simulink model "c_ff_pvcm_2dof_ax1_2"  (R2024b)
settings: Solver=VariableStepAuto  StartTime=0.0  StopTime=10.0  RelTol=1e-3
values from neighbouring files (symbols this model uses):
  Ct = 2.0e8    (= 200000000)    [check_2dof_model.m]    (also in ex9.m = 210000000; load_ex9_model.m)
  Dr = 0    [check_2dof_model.m]    (also in ex8_4.m; ex9.m; load_ex9_model.m)
  FBtype = 1    [check_2dof_model.m]    (also in ex8_4.m; ex9.m = -1; load_ex9_model.m)
  Jr = 3.0e-2    (= 0.03)    [check_2dof_model.m]    (also in ex9.m; load_ex9_model.m; load_params.m = 0.00222)
  Kpp = 40    [check_2dof_model.m]    (also in ex8_4.m = 4; ex9.m; load_ex9_model.m)
  KT = 1    [check_2dof_model.m]    (also in ex8_4.m; ex9.m; load_ex9_model.m)
  Kt = 1.0e8    (= 100000000)    [check_2dof_model.m]    (also in ex9.m; load_ex9_model.m; load_params.m = 110000000)
  Kvf = 0.7    [check_2dof_model.m]    (also in ex9.m; load_ex9_model.m)
  Kvi = 60    [check_2dof_model.m]    (also in ex8_4.m = 80; ex9.m = 63; load_ex9_model.m)
  Kvp = (Ja*Wvc)/KT    (= 7.26079271019)    [check_2dof_model.m]    (also in ex8_4.m = Ja*Wvc/KT; ex9.m = 7.62383234569; load_ex9_model.m)
  Mt = 100    [check_2dof_model.m]    (also in ex9.m = 200; load_ex9_model.m; load_params.m = 500)
  pfb_on = 1    [check_2dof_model.m]    (also in ex8_4.m; ex9.m; load_ex9_model.m)
  R = lp/2/pi    (= 0.00159154943092)    [check_2dof_model.m]    (also in ex9.m; load_ex9_model.m; load_params.m = 0.0032)
  vfb_on = 1    [check_2dof_model.m]    (also in ex8_4.m; ex9.m; load_ex9_model.m)
settings Model: Creator=shohei  LastModifiedBy=shohei

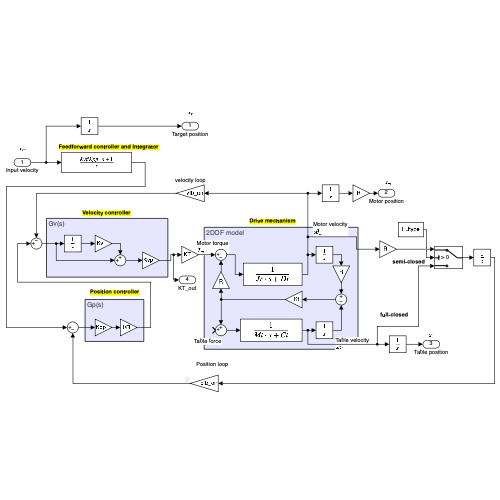
[thumbnail: Simulink's stored preview of the top-level diagram]
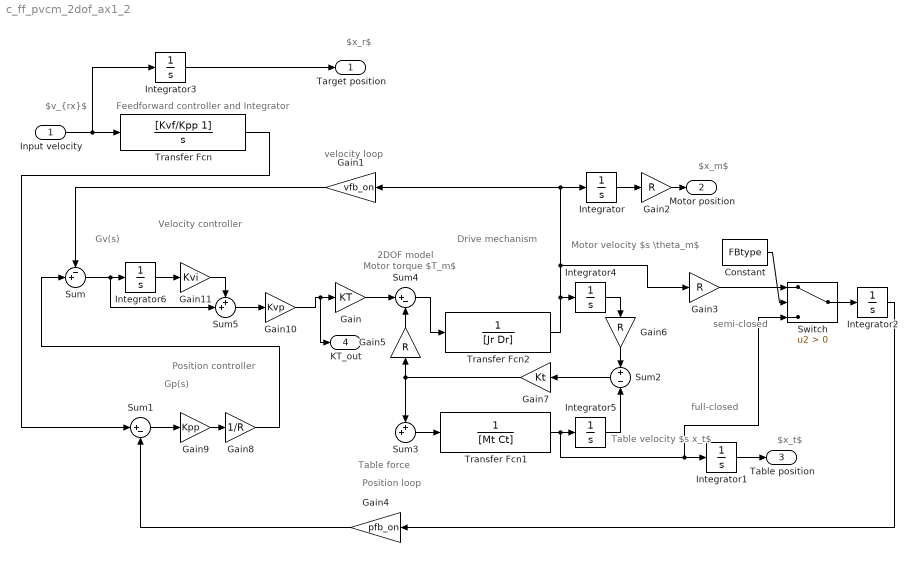
== system c_ff_pvcm_2dof_ax1_2 ==
  note: Gv(s)
  note: Gp(s)
  note: 2DOF model
  note: $v_{rx}$
  note: $x_r$
  note: $x_t$
  note: Velocity controller
  note: Drive mechanism
  note: Position controller
  note: velocity loop
  note: semi-closed
  note: full-closed
  note: Position loop
  note: Feedforward controller and Integrator
  note: $x_m$
  note: Motor velocity
      | $s \theta_m$
  note: Table velocity
      | $s x_t$
  note: Motor torque
      | $T_m$
  note: Table force
  Input velocity : Inport
  Constant : Constant  Value=FBtype
  Gain : Gain  Gain=KT
  Gain1 : Gain  Gain=vfb_on
  Gain10 : Gain  Gain=Kvp
  Gain11 : Gain  Gain=Kvi
  Gain{2..3,5..6} (4 alike) : Gain  Gain=R
  Gain4 : Gain  Gain=pfb_on
  Gain7 : Gain  Gain=Kt
  Gain8 : Gain  Gain=1/R
  Gain9 : Gain  Gain=Kpp
  Integrator{,1..6} (7 alike) : Integrator
  Sum : Sum  Inputs=-+|
  Sum1 : Sum  Inputs=|+-
  Sum2 : Sum  Inputs=+|-
  Sum3 : Sum  Inputs=++|
  Sum4 : Sum  Inputs=|+-
  Sum5 : Sum  Inputs=++|
  Switch : Switch  Criteria=u2 > Threshold  SaturateOnIntegerOverflow=off  InputSameDT=off
  Transfer Fcn : TransferFcn  Numerator=[Kvf/Kpp 1]  Denominator=[1 0]
  Transfer Fcn1 : TransferFcn  Denominator=[Mt Ct]
  Transfer Fcn2 : TransferFcn  Denominator=[Jr Dr]
  Target position : Outport
  Motor position : Outport  Port=2
  Table position : Outport  Port=3
  KT_out : Outport  Port=4
  wires:
  Gain8/1 -> Sum/2
  Switch/1 -> Integrator2/1
  Integrator1/1 -> Table position/1
  Integrator/1 -> Gain2/1
  Gain3/1 -> Switch/1
  Gain2/1 -> Motor position/1
  Transfer Fcn1/1 -> Integrator1/1, Switch/3, Integrator5/1
  Transfer Fcn2/1 -> Integrator/1, Gain1/1, Gain3/1, Integrator4/1
  Integrator2/1 -> Gain4/1
  Gain10/1 -> KT_out/1, Gain/1
  Constant/1 -> Switch/2
  Gain4/1 -> Sum1/2
  Gain1/1 -> Sum/1
  Integrator3/1 -> Target position/1
  Transfer Fcn/1 -> Sum1/1
  Input velocity/1 -> Integrator3/1, Transfer Fcn/1
  Gain7/1 -> Sum3/1, Gain5/1
  Sum4/1 -> Transfer Fcn2/1
  Gain/1 -> Sum4/1
  Integrator5/1 -> Sum2/2
  Sum2/1 -> Gain7/1
  Sum3/1 -> Transfer Fcn1/1
  Gain6/1 -> Sum2/1
  Gain5/1 -> Sum4/2
  Integrator4/1 -> Gain6/1
  Sum1/1 -> Gain9/1
  Gain9/1 -> Gain8/1
  Gain11/1 -> Sum5/1
  Sum5/1 -> Gain10/1
  Sum/1 -> Sum5/2, Integrator6/1
  Integrator6/1 -> Gain11/1
